simulink model "zad1_test"  (R2014b)
settings: Solver=ode45  StartTime=0.0  StopTime=1.75  RelTol=1e-3
settings Model: Creator=kuba  LastModifiedBy=kuba
settings DebuggingCC: SolverPrmCheckMsg=none

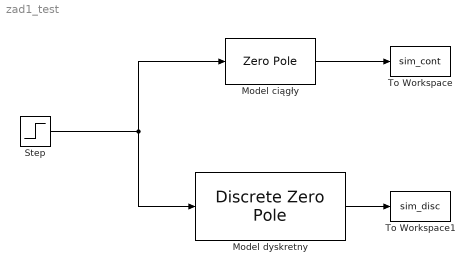
== system zad1_test ==
  Model ciągły : ZeroPole  Zeros=[-2.5 -7]  Poles=[8 -9 -10]
  Model dyskretny : DiscreteZeroPole  Zeros=[0.644 0.1554]  Poles=[7.389 0.105 0.082]  Gain=0.4496  SampleTime=0.25
  Step : Step  SampleTime=0
  To Workspace : ToWorkspace  VariableName=sim_cont  SaveFormat=Timeseries  SampleTime=-1
  To Workspace1 : ToWorkspace  VariableName=sim_disc  SaveFormat=Timeseries  SampleTime=-1
  wires:
  Model ciągły/1 -> To Workspace/1
  Model dyskretny/1 -> To Workspace1/1
  Step/1 -> Model ciągły/1, Model dyskretny/1
